simulink model "raibert_controller_1_1"  (R2018b)
settings: Solver=ode15s  StartTime=0.0  StopTime=inf  FixedStep=sample_time  MaxStep=1e-2  RelTol=1e-3
InitFcn:
  | addpath('../common/')
  | colors
  | addpath('functions/')
  | simulation_params
  | mechanical_params
StartFcn:
  | clc
  | tic
StopFcn:
  | stopscript
values from neighbouring files (symbols this model uses):
  sample_time = 1/sample_freq    (= 0.001)    [simulation_params.m]
undefined symbols (not defined in the file or in its folder): ctrl, sm
libraries: powerlib_meascontrol x1
settings Model: Creator=William  LastModifiedBy=akhadke
settings DataIOCC: SaveOutput=off  SaveTime=off
settings OptimizationCC: BlockReduction=off  DefaultParameterBehavior=Inlined  UseFloatMulNetSlope=on  InlineInvariantSignals=on  OptimizeBlockIOStorage=off  BufferReuse=off  GlobalBufferReuse=off  ExpressionFolding=off  LocalBlockOutputs=off  LifeSpan=0.5  SimCompilerOptimization=on  OptimizeDataStoreBuffers=off  BusAssignmentInplaceUpdate=off
settings DebuggingCC: UnderspecifiedInitializationDetection=Classic  MergeDetectMultiDrivingBlocksExec=none  LibraryContextMissingDiagnostic=none
settings HardwareCC: ProdBitPerPointer=32  ProdBitPerSizeT=32  ProdBitPerPtrDiffT=32  ProdLargestAtomicFloat=None  ProdWordSize=32  ProdLongLongMode=on  ProdHWDeviceType=Generic->32-bit x86 compatible
settings ModelReferenceCC: PropagateSignalLabelsOutOfModel=off
settings SFSimCC: SimUseLocalCustomCode=off
settings RTWCC: SystemTargetFile=slrt.tlc  TLCOptions=-axPCModelStackSizeKB=1024  TemplateMakefile=slrt_default_tmf  Description=Simulink Real-Time  RTWUseLocalCustomCode=off  CodeExecutionProfiling=on  RTWCompilerOptimization=on
settings CodeAppCC: MaxIdLength=127  StateflowObjectComments=on
settings TargetCC: CodeReplacementLibrary=XPC_BLAS  ParMdlRefBuildCompliant=on  ConcurrentExecutionCompliant=on  GeneratePreprocessorConditionals=Use local settings  MatFileLogging=on  PreserveStateflowLocalDataDimensions=off  MATLABClassNameForMDSCustomization=xpcAperiodicCustomization
settings SimscapeCC: SimscapeNormalizeSystem=off

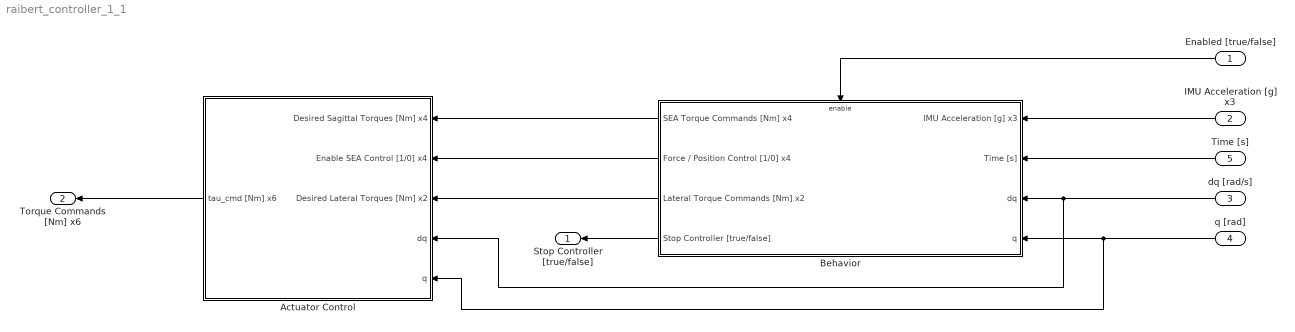
== system raibert_controller_1_1 ==
  Enabled [true/false] : Inport  OutDataTypeStr=boolean  PortDimensions=1  SampleTime=sample_time  Interpolate=off
  IMU Acceleration [g] x3 : Inport  Port=2  OutDataTypeStr=double  PortDimensions=3  SampleTime=[0.001,0]  Interpolate=off
  dq [rad/s] : Inport  Port=3  OutDataTypeStr=double  PortDimensions=13  SampleTime=[0.001,0]  Interpolate=off
  q [rad] : Inport  Port=4  OutDataTypeStr=double  PortDimensions=13  SampleTime=[0.001,0]  Interpolate=off
  Time [s] : Inport  Port=5  OutDataTypeStr=double  PortDimensions=1  SampleTime=sample_time  Interpolate=off
  Actuator Control : Subsystem
  Behavior : Subsystem
  Stop Controller [true/false] : Outport  OutDataTypeStr=boolean  PortDimensions=1  SampleTime=[0.001,0]  OutputWhenDisabled=reset  InitialOutput=[0 0 0 0 0 0]
  Torque Commands [Nm] x6 : Outport  Port=2  OutDataTypeStr=double  PortDimensions=6  SampleTime=[0.001,0]  OutputWhenDisabled=reset  InitialOutput=[0 0 0 0 0 0]
  wires:
  Behavior/2(Force / Position Control [1/0] x4) -> Actuator Control/2(Enable SEA Control [1/0] x4)
  IMU Acceleration [g] x3/1 -> Behavior/1(IMU Acceleration [g] x3)
  Time [s]/1 -> Behavior/2(Time [s])
  Behavior/3(Lateral Torque Commands [Nm] x2) -> Actuator Control/3(Desired Lateral Torques [Nm] x2)
  Behavior/1(SEA Torque Commands [Nm] x4) -> Actuator Control/1(Desired Sagittal Torques [Nm] x4)
  Actuator Control/1(tau_cmd [Nm] x6) -> Torque Commands [Nm] x6/1
  q [rad]/1 -> Actuator Control/5(q), Behavior/4(q)
  dq [rad/s]/1 -> Actuator Control/4(dq), Behavior/3(dq)
  Enabled [true/false]/1 -> Behavior/Enable
  Behavior/4(Stop Controller [true/false]) -> Stop Controller [true/false]/1

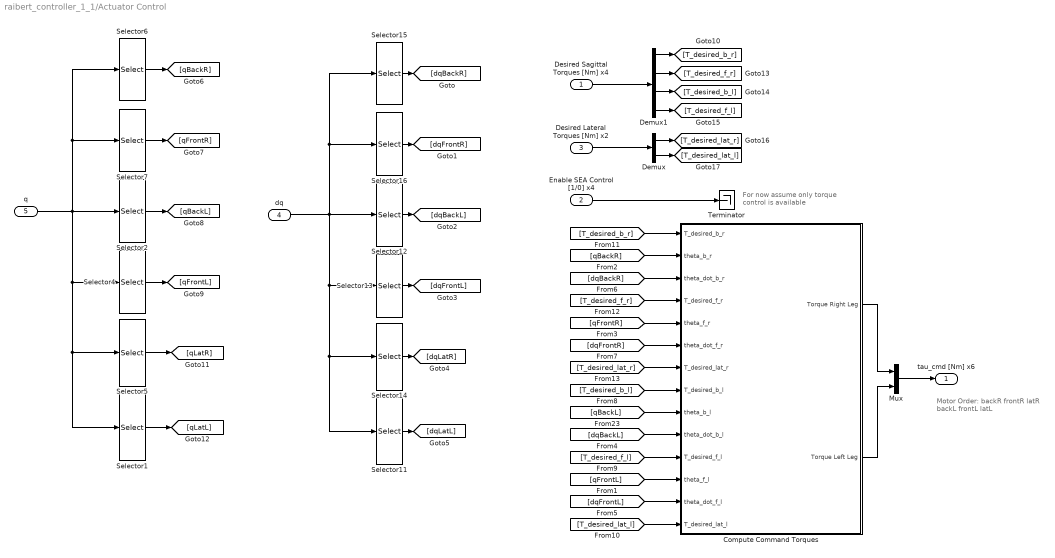
== system raibert_controller_1_1/Actuator Control ==
  note: Motor Order:
      |
      | backR
      | frontR
      | latR
      | backL
      | frontL
      | latL
  note: For now assume only
      | torque control is available
  Desired Sagittal Torques [Nm] x4 : Inport  OutDataTypeStr=double  PortDimensions=4  SampleTime=sample_time
  Enable SEA Control [1/0] x4 : Inport  Port=2  OutDataTypeStr=boolean  PortDimensions=4  SampleTime=sample_time
  Desired Lateral Torques [Nm] x2 : Inport  Port=3  OutDataTypeStr=double  PortDimensions=2  SampleTime=sample_time
  dq : Inport  Port=4  OutDataTypeStr=double  PortDimensions=13  SampleTime=sample_time
  q : Inport  Port=5  OutDataTypeStr=double  PortDimensions=13  SampleTime=sample_time
  Compute Command Torques : Subsystem
  Demux : Demux  Outputs=2
  Demux1 : Demux
  Mux : Mux  Inputs=2
  Selector1 : Selector  InputPortWidth=13  IndexOptions=Index vector (dialog)  Indices=[10]  OutputSizes=1
  Selector11 : Selector  InputPortWidth=13  IndexOptions=Index vector (dialog)  Indices=[10]  OutputSizes=1
  Selector12 : Selector  InputPortWidth=13  IndexOptions=Index vector (dialog)  Indices=[5 6]  OutputSizes=1
  Selector13 : Selector  InputPortWidth=13  IndexOptions=Index vector (dialog)  Indices=[7 8]  OutputSizes=1
  Selector14 : Selector  InputPortWidth=13  IndexOptions=Index vector (dialog)  Indices=[9]  OutputSizes=1
  Selector15 : Selector  InputPortWidth=13  IndexOptions=Index vector (dialog)  Indices=[1 2]  OutputSizes=1
  Selector16 : Selector  InputPortWidth=13  IndexOptions=Index vector (dialog)  Indices=[3 4]  OutputSizes=1
  Selector2 : Selector  InputPortWidth=13  IndexOptions=Index vector (dialog)  Indices=[5 6]  OutputSizes=1
  Selector4 : Selector  InputPortWidth=13  IndexOptions=Index vector (dialog)  Indices=[7 8]  OutputSizes=1
  Selector5 : Selector  InputPortWidth=13  IndexOptions=Index vector (dialog)  Indices=[9]  OutputSizes=1
  Selector6 : Selector  InputPortWidth=13  IndexOptions=Index vector (dialog)  Indices=[1 2]  OutputSizes=1
  Selector7 : Selector  InputPortWidth=13  IndexOptions=Index vector (dialog)  Indices=[3 4]  OutputSizes=1
  Terminator : Terminator
  tau_cmd [Nm] x6 : Outport  OutDataTypeStr=double  PortDimensions=6  InitialOutput=[0 0 0 0 0 0]
  wires:
  Compute Command Torques/2(Torque Left Leg) -> Mux/2
  Compute Command Torques/1(Torque Right Leg) -> Mux/1
  Mux/1 -> tau_cmd [Nm] x6/1
  [T_desired_lat_r] -> Compute Command Torques/7(T_desired_lat_r)
  [T_desired_f_r] -> Compute Command Torques/4(T_desired_f_r)
  [T_desired_b_r] -> Compute Command Torques/1(T_desired_b_r)
  Demux/2 -> [T_desired_lat_l]
  Demux/1 -> [T_desired_lat_r]
  [T_desired_lat_l] -> Compute Command Torques/14(T_desired_lat_l)
  [T_desired_f_l] -> Compute Command Torques/11(T_desired_f_l)
  [T_desired_b_l] -> Compute Command Torques/8(T_desired_b_l)
  Demux1/4 -> [T_desired_f_l]
  Demux1/3 -> [T_desired_b_l]
  Demux1/2 -> [T_desired_f_r]
  Demux1/1 -> [T_desired_b_r]
  Enable SEA Control [1/0] x4/1 -> Terminator/1
  Desired Sagittal Torques [Nm] x4/1 -> Demux1/1
  Desired Lateral Torques [Nm] x2/1 -> Demux/1
  [qBackR] -> Compute Command Torques/2(theta_b_r)
  [dqBackR] -> Compute Command Torques/3(theta_dot_b_r)
  [qFrontR] -> Compute Command Torques/5(theta_f_r)
  [dqFrontR] -> Compute Command Torques/6(theta_dot_f_r)
  [dqFrontL] -> Compute Command Torques/13(theta_dot_f_l)
  [qFrontL] -> Compute Command Torques/12(theta_f_l)
  [qBackL] -> Compute Command Torques/9(theta_b_l)
  [dqBackL] -> Compute Command Torques/10(theta_dot_b_l)
  Selector14/1 -> [dqLatR]
  Selector16/1 -> [dqFrontR]
  Selector7/1 -> [qFrontR]
  q/1 -> Selector2/1, Selector7/1, Selector6/1, Selector4/1, Selector5/1, Selector1/1
  Selector11/1 -> [dqLatL]
  dq/1 -> Selector11/1, Selector14/1, Selector13/1, Selector15/1, Selector16/1, Selector12/1
  Selector6/1 -> [qBackR]
  Selector5/1 -> [qLatR]
  Selector4/1 -> [qFrontL]
  Selector2/1 -> [qBackL]
  Selector12/1 -> [dqBackL]
  Selector1/1 -> [qLatL]
  Selector13/1 -> [dqFrontL]
  Selector15/1 -> [dqBackR]

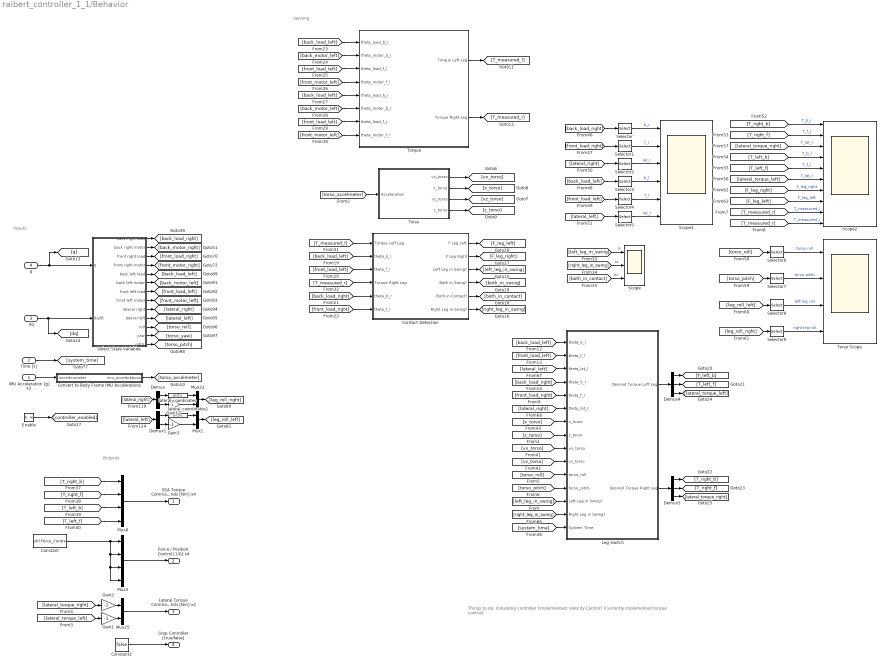
== system raibert_controller_1_1/Behavior ==
  note: Inputs
  note: Sensing
  note: Outputs
  note: Things to do:
      | Initializing controller (implemented)
      | Velocity Control? (Currently implemented torque control)
  IMU Acceleration [g] x3 : Inport  OutDataTypeStr=double  PortDimensions=3  SampleTime=[0.001,0]
  Time [s] : Inport  Port=2  OutDataTypeStr=double  PortDimensions=1  SampleTime=[0.001,0]
  dq : Inport  Port=3  OutDataTypeStr=double  PortDimensions=13  SampleTime=[0.001,0]
  q : Inport  Port=4  OutDataTypeStr=double  PortDimensions=13  SampleTime=[0.001,0]
  Enable : EnablePort  PropagateVarSize=During execution  ShowOutputPort=on
  Constant : Constant  Value=ctrl.Force_Control
  Constant2 : Constant  Value=false
  Contact Detection : Subsystem
  Convert to Body Frame IMU Accelerations : MATLAB Function  TreatAsAtomicUnit=on
  Demux : Demux  Outputs=2
  Demux1 : Demux  Outputs=2
  Demux3 : Demux  Outputs=3
  Demux4 : Demux  Outputs=3
  Gain{1..3,12} (4 alike) : Gain  Gain=-1
  Leg Switch : Subsystem
  Mux1 : Mux  Inputs=2
  Mux22 : Mux  Inputs=2
  Mux25 : Mux  Inputs=2
  Mux3 : Mux
  Mux8 : Mux
  Scope : Scope  NumInputPorts=3
  Scope1 : Scope  NumInputPorts=6
  Scope2 : Scope  NumInputPorts=10
  Select State Variables : Subsystem
  Selector{,1..9} (10 alike) : Selector  InputPortWidth=2  IndexOptions=Index vector (dialog)  Indices=[1]  OutputSizes=1
  Torque : Subsystem
  Torso : Subsystem
  Torso Scope : Scope  NumInputPorts=4
  lateral_coordinates : Fcn  Expr=pi/2-u
  lateral_coordinates1 : Fcn  Expr=pi/2-u
  SEA Torque Commands [Nm] x4 : Outport  OutDataTypeStr=double  PortDimensions=4  SampleTime=[0.001,0]  OutputWhenDisabled=reset  InitialOutput=[0 0 0 0]
  Force / Position Control [1/0] x4 : Outport  Port=2  OutDataTypeStr=boolean  PortDimensions=4  SampleTime=[0.001,0]  OutputWhenDisabled=reset  InitialOutput=[0 0 0 0]
  Lateral Torque Commands [Nm] x2 : Outport  Port=3  OutDataTypeStr=double  PortDimensions=2  SampleTime=[0.001,0]  OutputWhenDisabled=reset  InitialOutput=[0 0]
  Stop Controller [true/false] : Outport  Port=4  OutDataTypeStr=boolean  PortDimensions=1  SampleTime=[0.001,0]  OutputWhenDisabled=reset  InitialOutput=0
  wires:
  [T_measured_r] -> Scope2/10  "T_measured_r"
  [T_measured_r] -> Scope2/9  "T_measured_l"
  [torso_pitch] -> Leg Switch/12(torso_pitch)
  [torso_roll] -> Leg Switch/11(torso_roll)
  [z_torso] -> Leg Switch/8(z_torso)
  [x_torso] -> Leg Switch/7(x_torso)
  [vz_torso] -> Leg Switch/10(vz_torso)
  [vx_torso] -> Leg Switch/9(vx_torso)
  [lateral_right] -> Leg Switch/6(theta_lat_r)
  [lateral_left] -> Leg Switch/3(theta_lat_l)
  [right_leg_in_swing] -> Leg Switch/14(Right Leg in Swing?)
  [F_leg_left] -> Scope2/8  "F_leg_left"
  [F_leg_right] -> Scope2/7  "F_leg_right"
  Contact Detection/2(F Leg Right) -> [F_leg_right]
  Contact Detection/1(F Leg Left) -> [F_leg_left]
  [leg_roll_right] -> Selector9/1
  Selector9/1 -> Torso Scope/4  "right leg roll"
  [leg_roll_left] -> Selector8/1
  Selector8/1 -> Torso Scope/3  "left leg roll"
  [torso_pitch] -> Selector7/1
  Selector7/1 -> Torso Scope/2  "torso pitch"
  Selector6/1 -> Torso Scope/1  "torso roll"
  [torso_roll] -> Selector6/1
  [lateral_torque_left] -> Scope2/6  "T_lat_l"
  [lateral_torque_right] -> Scope2/3  "T_lat_r"
  [T_left_f] -> Scope2/5  "T_f_l"
  [T_left_b] -> Scope2/4  "T_b_l"
  [T_right_f] -> Scope2/2  "T_f_r"
  [T_right_b] -> Scope2/1  "T_b_r"
  [back_load_right] -> Selector/1
  Selector/1 -> Scope1/1  "b_r"
  Selector2/1 -> Scope1/3  "lat_r"
  [back_load_left] -> Selector3/1
  Selector5/1 -> Scope1/6  "lat_l"
  [lateral_left] -> Selector5/1
  [lateral_right] -> Selector2/1
  Selector4/1 -> Scope1/5  "f_l"
  [front_load_left] -> Selector4/1
  Selector3/1 -> Scope1/4  "b_l"
  [front_load_right] -> Selector1/1
  Selector1/1 -> Scope1/2  "f_r"
  Demux3/3 -> [lateral_torque_right]
  Demux3/2 -> [T_right_f]
  Demux3/1 -> [T_right_b]
  Demux4/3 -> [lateral_torque_left]
  [back_motor_left] -> Torque/6(theta_motor_b_r)
  [back_load_left] -> Torque/5(theta_load_b_r)
  [back_motor_left] -> Torque/2(theta_motor_b_l)
  [front_motor_left] -> Torque/8(theta_motor_f_r)
  [back_load_left] -> Torque/1(theta_load_b_l)
  Torque/2(Torque Right Leg) -> [T_measured_r]
  [front_motor_left] -> Torque/4(theta_motor_f_l)
  [front_load_left] -> Torque/7(theta_load_f_r)
  [front_load_left] -> Torque/3(theta_load_f_l)
  Torque/1(Torque Left Leg) -> [T_measured_l]
  [T_left_f] -> Mux8/4
  [T_left_b] -> Mux8/3
  [T_right_f] -> Mux8/2
  [T_right_b] -> Mux8/1
  Leg Switch/2(Desired Torque Right Leg) -> Demux3/1
  Leg Switch/1(Desired Torque Left Leg) -> Demux4/1
  Demux4/1 -> [T_left_b]
  Demux4/2 -> [T_left_f]
  [system_time] -> Leg Switch/15(System Time)
  Contact Detection/4(Both in Swing?) -> [both_in_swing]
  Contact Detection/5(Both in Contact?) -> [both_in_contact]
  Contact Detection/6(Right Leg in Swing?) -> [right_leg_in_swing]
  Contact Detection/3(Left Leg in Swing?) -> [left_leg_in_swing]
  [both_in_contact] -> Scope/3  "bc"
  [right_leg_in_swing] -> Scope/2  "rs"
  [left_leg_in_swing] -> Scope/1  "ls"
  [T_measured_r] -> Contact Detection/4(Torque Right Leg)
  [T_measured_l] -> Contact Detection/1(Torque Left Leg)
  [front_load_right] -> Contact Detection/6(theta_f_r)
  [back_load_right] -> Contact Detection/5(theta_b_r)
  [front_load_left] -> Contact Detection/3(theta_f_l)
  [back_load_left] -> Contact Detection/2(theta_b_l)
  Torso/4(z_torso) -> [z_torso]
  Torso/2(x_torso) -> [x_torso]
  Torso/3(vz_torso) -> [vz_torso]
  Torso/1(vx_torso) -> [vx_torso]
  [left_leg_in_swing] -> Leg Switch/13("Left Leg in Swing? ")
  Constant/1 -> Mux3/1, Mux3/2, Mux3/3, Mux3/4
  [front_load_left] -> Leg Switch/2(theta_f_l)
  [back_load_left] -> Leg Switch/1(theta_b_l)
  [front_load_right] -> Leg Switch/5(theta_f_r)
  [back_load_right] -> Leg Switch/4(theta_b_r)
  [torso_accelmeter] -> Torso/1(Acceleration)
  IMU Acceleration [g] x3/1 -> Convert to Body Frame IMU Accelerations/1(accelerometer)
  Convert to Body Frame IMU Accelerations/1(imu_accelerations) -> [torso_accelmeter]
  Enable/1 -> [controller_enabled]
  Demux1/2 -> Gain3/1
  lateral_coordinates1/1 -> Mux1/1
  Gain3/1 -> Mux1/2
  Mux1/1 -> [leg_roll_left]
  Demux1/1 -> lateral_coordinates1/1
  [lateral_left] -> Demux1/1
  [lateral_right] -> Demux/1
  Select State Variables/9(lateral right) -> [lateral_right]
  Select State Variables/10(lateral left) -> [lateral_left]
  Select State Variables/11(roll) -> [torso_roll]
  Select State Variables/12(yaw) -> [torso_yaw]
  Select State Variables/13(pitch) -> [torso_pitch]
  Select State Variables/8(front left motor) -> [front_motor_left]
  Select State Variables/7(front left load) -> [front_load_left]
  Select State Variables/6(back left motor) -> [back_motor_left]
  Select State Variables/5(back left load) -> [back_load_left]
  Select State Variables/4(front right motor) -> [front_motor_right]
  Select State Variables/3(front right load) -> [front_load_right]
  Select State Variables/2(back right motor) -> [back_motor_right]
  Select State Variables/1(back right load) -> [back_load_right]
  dq/1 -> Select State Variables/2(dq/dt), [dq]
  Constant2/1 -> Stop Controller [true/false]/1
  Gain1/1 -> Mux25/2
  Mux25/1 -> Lateral Torque Commands [Nm] x2/1
  Gain2/1 -> Mux25/1
  Mux3/1 -> Force / Position Control [1/0] x4/1
  Mux8/1 -> SEA Torque Commands [Nm] x4/1
  [lateral_torque_left] -> Gain1/1
  q/1 -> Select State Variables/1(q), [q]
  [lateral_torque_right] -> Gain2/1
  Demux/1 -> lateral_coordinates/1
  Mux22/1 -> [leg_roll_right]
  Gain12/1 -> Mux22/2
  lateral_coordinates/1 -> Mux22/1
  Demux/2 -> Gain12/1
  Time [s]/1 -> [system_time]

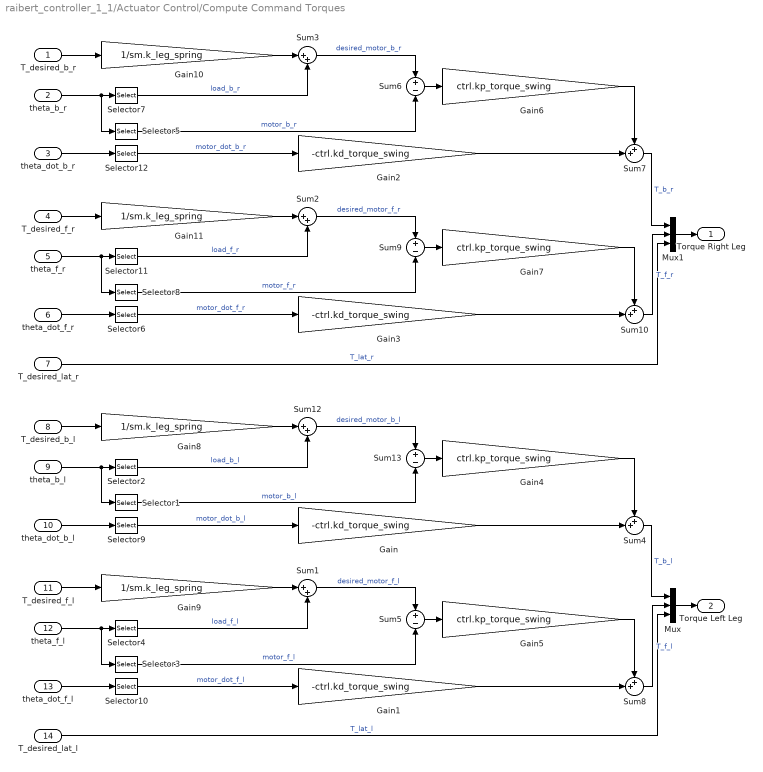
== system raibert_controller_1_1/Actuator Control/Compute Command Torques ==
  T_desired_b_r : Inport
  theta_b_r : Inport  Port=2
  theta_dot_b_r : Inport  Port=3
  T_desired_f_r : Inport  Port=4
  theta_f_r : Inport  Port=5
  theta_dot_f_r : Inport  Port=6
  T_desired_lat_r : Inport  Port=7
  T_desired_b_l : Inport  Port=8
  theta_b_l : Inport  Port=9
  theta_dot_b_l : Inport  Port=10
  T_desired_f_l : Inport  Port=11
  theta_f_l : Inport  Port=12
  theta_dot_f_l : Inport  Port=13
  T_desired_lat_l : Inport  Port=14
  Gain{,1..3} (4 alike) : Gain  Gain=-ctrl.kd_torque_swing
  Gain{8..11} (4 alike) : Gain  Gain=1/sm.k_leg_spring
  Gain{4..7} (4 alike) : Gain  Gain=ctrl.kp_torque_swing
  Mux : Mux  Inputs=3
  Mux1 : Mux  Inputs=3
  Selector{1,3,5..6,8..10,12} (8 alike) : Selector  InputPortWidth=2  IndexOptions=Index vector (dialog)  Indices=[2]  OutputSizes=1
  Selector{2,4,7,11} (4 alike) : Selector  InputPortWidth=2  IndexOptions=Index vector (dialog)  Indices=[1]  OutputSizes=1
  Sum{1..3,12} (4 alike) : Sum  Inputs=|++
  Sum{4,7..8,10} (4 alike) : Sum  Inputs=++|
  Sum{5..6,9,13} (4 alike) : Sum  Inputs=+-
  Torque Right Leg : Outport
  Torque Left Leg : Outport  Port=2
  wires:
  Sum9/1 -> Gain7/1
  theta_f_r/1 -> Selector11/1, Selector8/1
  Selector8/1 -> Sum9/2  "motor_f_r"
  T_desired_f_r/1 -> Gain11/1
  Gain11/1 -> Sum2/1
  Selector5/1 -> Sum6/2  "motor_b_r"
  theta_dot_b_r/1 -> Selector12/1
  Gain3/1 -> Sum10/2
  Selector12/1 -> Gain2/1  "motor_dot_b_r"
  Gain6/1 -> Sum7/1
  Gain2/1 -> Sum7/2
  Mux1/1 -> Torque Right Leg/1
  Selector6/1 -> Gain3/1  "motor_dot_f_r"
  Sum3/1 -> Sum6/1  "desired_motor_b_r"
  T_desired_lat_r/1 -> Mux1/3  "T_lat_r"
  T_desired_b_r/1 -> Gain10/1
  theta_b_r/1 -> Selector7/1, Selector5/1
  theta_dot_f_r/1 -> Selector6/1
  Sum2/1 -> Sum9/1  "desired_motor_f_r"
  Gain10/1 -> Sum3/1
  Gain7/1 -> Sum10/1
  Selector7/1 -> Sum3/2  "load_b_r"
  Sum7/1 -> Mux1/1  "T_b_r"
  Sum6/1 -> Gain6/1
  Selector11/1 -> Sum2/2  "load_f_r"
  Sum10/1 -> Mux1/2  "T_f_r"
  T_desired_lat_l/1 -> Mux/3  "T_lat_l"
  Sum8/1 -> Mux/2  "T_f_l"
  T_desired_f_l/1 -> Gain9/1
  theta_f_l/1 -> Selector4/1, Selector3/1
  Sum1/1 -> Sum5/1  "desired_motor_f_l"
  Selector3/1 -> Sum5/2  "motor_f_l"
  Gain9/1 -> Sum1/1
  Gain1/1 -> Sum8/2
  theta_dot_f_l/1 -> Selector10/1
  Selector10/1 -> Gain1/1  "motor_dot_f_l"
  Gain5/1 -> Sum8/1
  Selector4/1 -> Sum1/2  "load_f_l"
  Sum5/1 -> Gain5/1
  Gain4/1 -> Sum4/1
  Gain/1 -> Sum4/2
  Sum13/1 -> Gain4/1
  Sum12/1 -> Sum13/1  "desired_motor_b_l"
  Gain8/1 -> Sum12/1
  T_desired_b_l/1 -> Gain8/1
  theta_dot_b_l/1 -> Selector9/1
  Selector9/1 -> Gain/1  "motor_dot_b_l"
  theta_b_l/1 -> Selector2/1, Selector1/1
  Selector2/1 -> Sum12/2  "load_b_l"
  Selector1/1 -> Sum13/2  "motor_b_l"
  Sum4/1 -> Mux/1  "T_b_l"
  Mux/1 -> Torque Left Leg/1

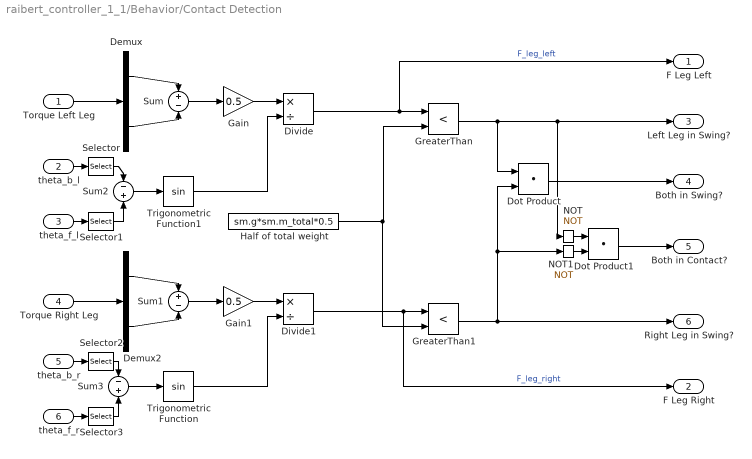
== system raibert_controller_1_1/Behavior/Contact Detection ==
  Torque Left Leg : Inport
  theta_b_l : Inport  Port=2
  theta_f_l : Inport  Port=3
  Torque Right Leg : Inport  Port=4
  theta_b_r : Inport  Port=5
  theta_f_r : Inport  Port=6
  Demux : Demux  Outputs=2
  Demux2 : Demux  Outputs=2
  Divide : Product  Inputs=*/
  Divide1 : Product  Inputs=*/
  Dot Product : DotProduct  InputSameDT=on  OutDataTypeStr=Inherit: Inherit via internal rule
  Dot Product1 : DotProduct  InputSameDT=on  OutDataTypeStr=Inherit: Inherit via internal rule
  Gain : Gain  Gain=0.5
  Gain1 : Gain  Gain=0.5
  GreaterThan : RelationalOperator  Operator=<  OutDataTypeStr=boolean  RndMeth=Simplest
  GreaterThan1 : RelationalOperator  Operator=<  OutDataTypeStr=boolean  RndMeth=Simplest
  Half of total weight : Constant  Value=sm.g*sm.m_total*0.5
  NOT : Logic  Operator=NOT  IconShape=distinctive  AllPortsSameDT=off  OutDataTypeStr=boolean
  NOT1 : Logic  Operator=NOT  IconShape=distinctive  AllPortsSameDT=off  OutDataTypeStr=boolean
  Selector{,1..3} (4 alike) : Selector  InputPortWidth=2  IndexOptions=Index vector (dialog)  Indices=[1]  OutputSizes=1
  Sum : Sum  Inputs=+-
  Sum1 : Sum  Inputs=+-
  Sum2 : Sum  Inputs=-+
  Sum3 : Sum  Inputs=-+
  Trigonometric Function : Trigonometry
  Trigonometric Function1 : Trigonometry
  F Leg Left : Outport
  F Leg Right : Outport  Port=2
  Left Leg in Swing? : Outport  Port=3
  Both in Swing? : Outport  Port=4
  Both in Contact? : Outport  Port=5
  Right Leg in Swing? : Outport  Port=6
  wires:
  Selector3/1 -> Sum3/2
  Selector2/1 -> Sum3/1
  Selector1/1 -> Sum2/2
  Selector/1 -> Sum2/1
  NOT1/1 -> Dot Product1/2
  NOT/1 -> Dot Product1/1
  Dot Product1/1 -> Both in Contact?/1
  Dot Product/1 -> Both in Swing?/1
  GreaterThan1/1 -> Right Leg in Swing?/1, Dot Product/2, NOT1/1
  GreaterThan/1 -> Left Leg in Swing?/1, NOT/1, Dot Product/1
  Half of total weight/1 -> GreaterThan/2, GreaterThan1/2
  Divide1/1 -> GreaterThan1/1, F Leg Right/1  "F_leg_right"
  Divide/1 -> GreaterThan/1, F Leg Left/1  "F_leg_left"
  Trigonometric Function/1 -> Divide1/2
  Gain1/1 -> Divide1/1
  Trigonometric Function1/1 -> Divide/2
  Gain/1 -> Divide/1
  Sum2/1 -> Trigonometric Function1/1
  Sum3/1 -> Trigonometric Function/1
  theta_b_r/1 -> Selector2/1
  theta_f_r/1 -> Selector3/1
  theta_b_l/1 -> Selector/1
  theta_f_l/1 -> Selector1/1
  Sum1/1 -> Gain1/1
  Sum/1 -> Gain/1
  Demux2/2 -> Sum1/2
  Demux2/1 -> Sum1/1
  Torque Right Leg/1 -> Demux2/1
  Demux/2 -> Sum/2
  Demux/1 -> Sum/1
  Torque Left Leg/1 -> Demux/1

== system raibert_controller_1_1/Behavior/Leg Switch ==
  theta_b_l : Inport
  theta_f_l : Inport  Port=2
  theta_lat_l : Inport  Port=3
  theta_b_r : Inport  Port=4
  theta_f_r : Inport  Port=5
  theta_lat_r : Inport  Port=6
  x_torso : Inport  Port=7
  z_torso : Inport  Port=8
  vx_torso : Inport  Port=9
  vz_torso : Inport  Port=10
  torso_roll : Inport  Port=11
  torso_pitch : Inport  Port=12
  "Left Leg in Swing? " : Inport  Port=13
  Right Leg in Swing? : Inport  Port=14
  System Time : Inport  Port=15
  Initialization Controller : Subsystem
  Logical Operator : Logic  AllPortsSameDT=off  OutDataTypeStr=boolean
  NOT : Logic  Operator=NOT  IconShape=distinctive  AllPortsSameDT=off  OutDataTypeStr=boolean
  Raibert : Subsystem
  Sum : Sum  Inputs=|++
  Sum1 : Sum  Inputs=|++
  Desired Torque Left Leg : Outport  SampleTime=[0.001, 0]
  Desired Torque Right Leg : Outport  Port=2  SampleTime=[0.001 0]
  wires:
  vz_torso/1 -> Raibert/10(vz_torso)
  torso_roll/1 -> Raibert/11(torso_roll)
  torso_pitch/1 -> Raibert/12(torso_pitch)
  vx_torso/1 -> Raibert/9(vx_torso)
  z_torso/1 -> Raibert/8(z_torso)
  x_torso/1 -> Raibert/7(x_torso)
  Initialization Controller/2(Desired Torque Right Leg) -> Sum1/2
  Initialization Controller/1(Desired Torque Left Leg) -> Sum/2
  Sum1/1 -> Desired Torque Right Leg/1
  Sum/1 -> Desired Torque Left Leg/1
  theta_lat_r/1 -> Initialization Controller/6(theta_lat_r)
  theta_lat_l/1 -> Initialization Controller/3(theta_lat_l)
  NOT/1 -> Raibert/Enable
  Logical Operator/1 -> NOT/1, Initialization Controller/Enable
  Right Leg in Swing?/1 -> Logical Operator/1
  Raibert/2(Desired Torque Right Leg) -> Sum1/1
  Raibert/1(Desired Torque Left Leg) -> Sum/1
  theta_f_r/1 -> Raibert/6(theta_f_r), Initialization Controller/5(theta_f_r)
  theta_b_r/1 -> Raibert/5(theta_b_r), Initialization Controller/4(theta_b_r)
  theta_f_l/1 -> Raibert/4(theta_f_l), Initialization Controller/2(theta_f_l)
  theta_b_l/1 -> Raibert/3(theta_b_l), Initialization Controller/1(theta_b_l)
  System Time/1 -> Raibert/2(System Time)
  "Left Leg in Swing? "/1 -> Logical Operator/2, Raibert/1(Left Leg in Swing?)

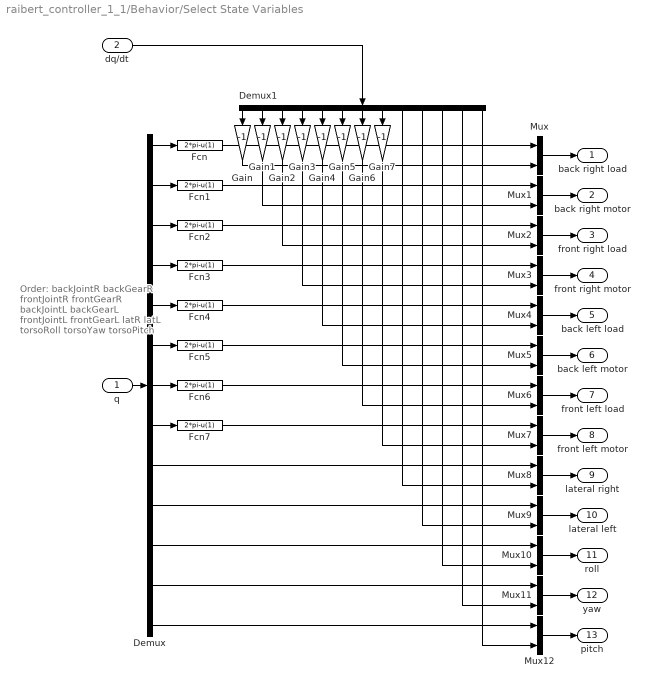
== system raibert_controller_1_1/Behavior/Select State Variables ==
  note: Order:
      |
      | backJointR
      | backGearR
      | frontJointR
      | frontGearR
      |
      | backJointL
      | backGearL
      | frontJointL
      | frontGearL
      |
      | latR
      | latL
      |
      | torsoRoll
      | torsoYaw
      | torsoPitch
  q : Inport
  dq/dt : Inport  Port=2
  Demux : Demux  Outputs=13
  Demux1 : Demux  Outputs=13
  Fcn{,1..7} (8 alike) : Fcn  Expr=2*pi-u(1)
  Gain{,1..7} (8 alike) : Gain  Gain=-1
  Mux{,1..12} (13 alike) : Mux  Inputs=2
  back right load : Outport
  back right motor : Outport  Port=2
  front right load : Outport  Port=3
  front right motor : Outport  Port=4
  back left load : Outport  Port=5
  back left motor : Outport  Port=6
  front left load : Outport  Port=7
  front left motor : Outport  Port=8
  lateral right : Outport  Port=9
  lateral left : Outport  Port=10
  roll : Outport  Port=11
  yaw : Outport  Port=12
  pitch : Outport  Port=13
  wires:
  Gain7/1 -> Mux7/2
  Gain6/1 -> Mux6/2
  Gain5/1 -> Mux5/2
  Gain4/1 -> Mux4/2
  Gain3/1 -> Mux3/2
  Gain2/1 -> Mux2/2
  Gain1/1 -> Mux1/2
  Gain/1 -> Mux/2
  Demux/9 -> Mux8/1
  Fcn7/1 -> Mux7/1
  Fcn6/1 -> Mux6/1
  Fcn5/1 -> Mux5/1
  Fcn4/1 -> Mux4/1
  Fcn3/1 -> Mux3/1
  Fcn2/1 -> Mux2/1
  Fcn1/1 -> Mux1/1
  Fcn/1 -> Mux/1
  dq/dt/1 -> Demux1/1
  Demux1/13 -> Mux12/2
  Demux1/12 -> Mux11/2
  Demux1/11 -> Mux10/2
  Demux1/10 -> Mux9/2
  Demux1/9 -> Mux8/2
  Demux1/8 -> Gain7/1
  Demux1/7 -> Gain6/1
  Demux1/6 -> Gain5/1
  Demux1/5 -> Gain4/1
  Demux1/4 -> Gain3/1
  Demux1/3 -> Gain2/1
  Demux1/2 -> Gain1/1
  Demux/13 -> Mux12/1
  Demux/12 -> Mux11/1
  Demux/11 -> Mux10/1
  Demux/10 -> Mux9/1
  Demux/8 -> Fcn7/1
  Demux/7 -> Fcn6/1
  Demux/6 -> Fcn5/1
  Demux/5 -> Fcn4/1
  Demux/4 -> Fcn3/1
  Demux/3 -> Fcn2/1
  Demux/2 -> Fcn1/1
  Demux1/1 -> Gain/1
  Demux/1 -> Fcn/1
  Mux11/1 -> yaw/1
  Mux10/1 -> roll/1
  Mux7/1 -> front left motor/1
  Mux6/1 -> front left load/1
  Mux3/1 -> front right motor/1
  Mux2/1 -> front right load/1
  Mux12/1 -> pitch/1
  Mux9/1 -> lateral left/1
  Mux8/1 -> lateral right/1
  Mux5/1 -> back left motor/1
  Mux4/1 -> back left load/1
  Mux1/1 -> back right motor/1
  Mux/1 -> back right load/1
  q/1 -> Demux/1

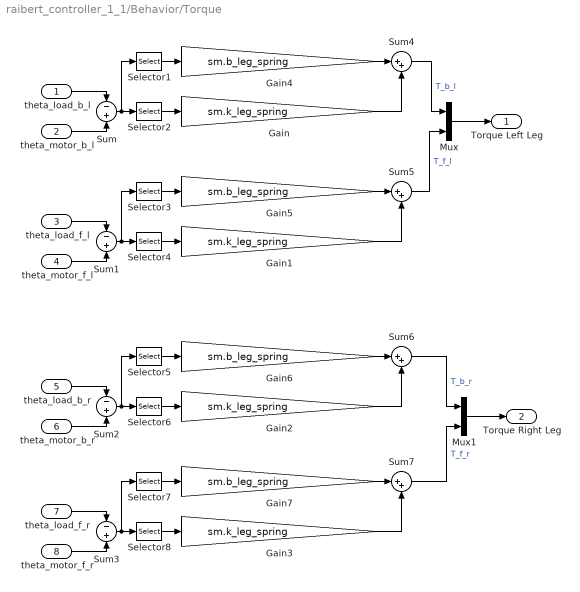
== system raibert_controller_1_1/Behavior/Torque ==
  theta_load_b_l : Inport
  theta_motor_b_l : Inport  Port=2
  theta_load_f_l : Inport  Port=3
  theta_motor_f_l : Inport  Port=4
  theta_load_b_r : Inport  Port=5
  theta_motor_b_r : Inport  Port=6
  theta_load_f_r : Inport  Port=7
  theta_motor_f_r : Inport  Port=8
  Gain{,1..3} (4 alike) : Gain  Gain=sm.k_leg_spring
  Gain{4..7} (4 alike) : Gain  Gain=sm.b_leg_spring
  Mux : Mux  Inputs=2
  Mux1 : Mux  Inputs=2
  Selector{1,3,5,7} (4 alike) : Selector  InputPortWidth=2  IndexOptions=Index vector (dialog)  Indices=[2]  OutputSizes=1
  Selector{2,4,6,8} (4 alike) : Selector  InputPortWidth=2  IndexOptions=Index vector (dialog)  Indices=[1]  OutputSizes=1
  Sum{,1..3} (4 alike) : Sum  Inputs=-+
  Sum{4..7} (4 alike) : Sum  Inputs=|++
  Torque Left Leg : Outport
  Torque Right Leg : Outport  Port=2
  wires:
  Selector8/1 -> Gain3/1
  Selector7/1 -> Gain7/1
  Sum3/1 -> Selector8/1, Selector7/1
  Selector6/1 -> Gain2/1
  Selector5/1 -> Gain6/1
  Sum2/1 -> Selector5/1, Selector6/1
  Selector3/1 -> Gain5/1
  Selector4/1 -> Gain1/1
  Sum1/1 -> Selector3/1, Selector4/1
  Selector1/1 -> Gain4/1
  Selector2/1 -> Gain/1
  Sum/1 -> Selector2/1, Selector1/1
  Sum7/1 -> Mux1/2  "T_f_r"
  Gain7/1 -> Sum7/1
  Gain3/1 -> Sum7/2
  Sum6/1 -> Mux1/1  "T_b_r"
  Gain6/1 -> Sum6/1
  Gain2/1 -> Sum6/2
  Sum5/1 -> Mux/2  "T_f_l"
  Gain5/1 -> Sum5/1
  Sum4/1 -> Mux/1  "T_b_l"
  Gain4/1 -> Sum4/1
  theta_motor_f_r/1 -> Sum3/2
  theta_load_f_r/1 -> Sum3/1
  Mux1/1 -> Torque Right Leg/1
  theta_motor_b_r/1 -> Sum2/2
  theta_load_b_r/1 -> Sum2/1
  Mux/1 -> Torque Left Leg/1
  theta_load_f_l/1 -> Sum1/1
  theta_motor_f_l/1 -> Sum1/2
  Gain1/1 -> Sum5/2
  Gain/1 -> Sum4/2
  theta_load_b_l/1 -> Sum/1
  theta_motor_b_l/1 -> Sum/2

== system raibert_controller_1_1/Behavior/Torso ==
  note: Things to do:
      | Add filtering?
  Acceleration : Inport
  "Integrator, Second-Order" : SecondOrderIntegrator  ICX=0
  "Integrator, Second-Order1" : SecondOrderIntegrator  ICX=sm.initial_com_height
  x : Selector  InputPortWidth=3  IndexOptions=Index vector (dialog)  Indices=[1]  OutputSizes=1
  z : Selector  InputPortWidth=3  IndexOptions=Index vector (dialog)  Indices=[3]  OutputSizes=1
  vx_torso : Outport
  x_torso : Outport  Port=2
  vz_torso : Outport  Port=3
  z_torso : Outport  Port=4
  wires:
  "Integrator, Second-Order1"/1 -> z_torso/1
  "Integrator, Second-Order"/1 -> x_torso/1
  "Integrator, Second-Order"/2 -> vx_torso/1
  "Integrator, Second-Order1"/2 -> vz_torso/1
  z/1 -> "Integrator, Second-Order1"/1
  x/1 -> "Integrator, Second-Order"/1
  Acceleration/1 -> x/1, z/1

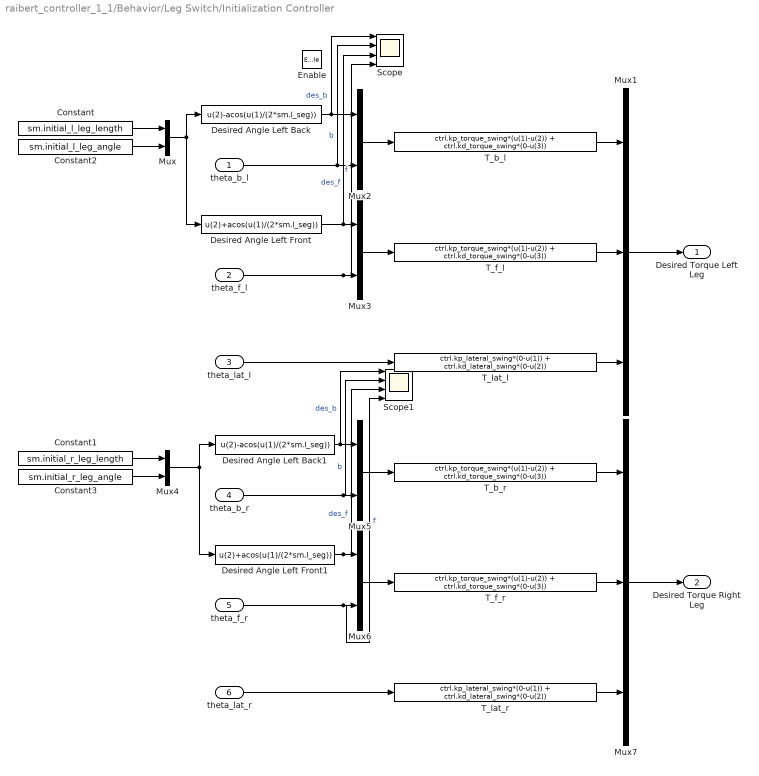
== system raibert_controller_1_1/Behavior/Leg Switch/Initialization Controller ==
  theta_b_l : Inport
  theta_f_l : Inport  Port=2
  theta_lat_l : Inport  Port=3
  theta_b_r : Inport  Port=4
  theta_f_r : Inport  Port=5
  theta_lat_r : Inport  Port=6
  Enable : EnablePort  StatesWhenEnabling=reset  PropagateVarSize=During execution
  Constant : Constant  Value=sm.initial_l_leg_length
  Constant1 : Constant  Value=sm.initial_r_leg_length
  Constant2 : Constant  Value=sm.initial_l_leg_angle
  Constant3 : Constant  Value=sm.initial_r_leg_angle
  Desired Angle Left Back : Fcn  Expr=u(2)-acos(u(1)/(2*sm.l_seg))
  Desired Angle Left Back1 : Fcn  Expr=u(2)-acos(u(1)/(2*sm.l_seg))
  Desired Angle Left Front : Fcn  Expr=u(2)+acos(u(1)/(2*sm.l_seg))
  Desired Angle Left Front1 : Fcn  Expr=u(2)+acos(u(1)/(2*sm.l_seg))
  Mux{,2..6} (6 alike) : Mux  Inputs=2
  Mux1 : Mux  Inputs=3
  Mux7 : Mux  Inputs=3
  Scope : Scope  NumInputPorts=4
  Scope1 : Scope  NumInputPorts=4
  T_b_l : Fcn  Expr=ctrl.kp_torque_swing*(u(1)-u(2)) + ctrl.kd_torque_swing*(0-u(3))
  T_b_r : Fcn  Expr=ctrl.kp_torque_swing*(u(1)-u(2)) + ctrl.kd_torque_swing*(0-u(3))
  T_f_l : Fcn  Expr=ctrl.kp_torque_swing*(u(1)-u(2)) + ctrl.kd_torque_swing*(0-u(3))
  T_f_r : Fcn  Expr=ctrl.kp_torque_swing*(u(1)-u(2)) + ctrl.kd_torque_swing*(0-u(3))
  T_lat_l : Fcn  Expr=ctrl.kp_lateral_swing*(0-u(1)) + ctrl.kd_lateral_swing*(0-u(2))
  T_lat_r : Fcn  Expr=ctrl.kp_lateral_swing*(0-u(1)) + ctrl.kd_lateral_swing*(0-u(2))
  Desired Torque Left Leg : Outport  InitialOutput=[0 0 0]
  Desired Torque Right Leg : Outport  Port=2  InitialOutput=[0 0 0]
  wires:
  theta_b_r/1 -> Mux5/2, Scope1/2  "b"
  theta_f_r/1 -> Mux6/2, Scope1/4  "f"
  Desired Angle Left Front1/1 -> Mux6/1, Scope1/3  "des_f"
  Desired Angle Left Back1/1 -> Mux5/1, Scope1/1  "des_b"
  Mux1/1 -> Desired Torque Left Leg/1
  Mux7/1 -> Desired Torque Right Leg/1
  T_lat_r/1 -> Mux7/3
  T_f_r/1 -> Mux7/2
  T_b_r/1 -> Mux7/1
  T_lat_l/1 -> Mux1/3
  T_f_l/1 -> Mux1/2
  T_b_l/1 -> Mux1/1
  Constant3/1 -> Mux4/2
  Constant1/1 -> Mux4/1
  Mux6/1 -> T_f_r/1
  Mux5/1 -> T_b_r/1
  theta_lat_r/1 -> T_lat_r/1
  Mux4/1 -> Desired Angle Left Back1/1, Desired Angle Left Front1/1
  Desired Angle Left Front/1 -> Mux3/1, Scope/3  "des_f"
  Mux3/1 -> T_f_l/1
  theta_f_l/1 -> Mux3/2, Scope/4  "f"
  Mux2/1 -> T_b_l/1
  theta_b_l/1 -> Mux2/2, Scope/2  "b"
  Desired Angle Left Back/1 -> Mux2/1, Scope/1  "des_b"
  Constant2/1 -> Mux/2
  Constant/1 -> Mux/1
  Mux/1 -> Desired Angle Left Back/1, Desired Angle Left Front/1
  theta_lat_l/1 -> T_lat_l/1

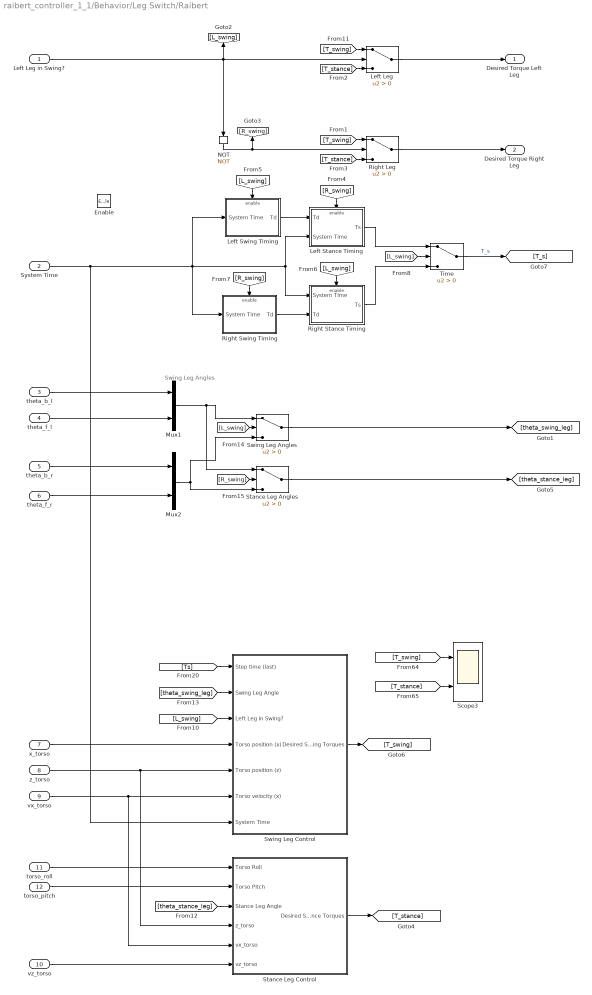
== system raibert_controller_1_1/Behavior/Leg Switch/Raibert ==
  note: Swing Leg Angles
  Left Leg in Swing? : Inport
  System Time : Inport  Port=2
  theta_b_l : Inport  Port=3
  theta_f_l : Inport  Port=4
  theta_b_r : Inport  Port=5
  theta_f_r : Inport  Port=6
  x_torso : Inport  Port=7
  z_torso : Inport  Port=8
  vx_torso : Inport  Port=9
  vz_torso : Inport  Port=10
  torso_roll : Inport  Port=11
  torso_pitch : Inport  Port=12
  Enable : EnablePort  StatesWhenEnabling=reset  PropagateVarSize=During execution
  Left Leg : Switch  Criteria=u2 > Threshold
  Left Stance Timing : Subsystem
  Left Swing Timing : Subsystem
  Mux1 : Mux  Inputs=2
  Mux2 : Mux  Inputs=2
  NOT : Logic  Operator=NOT  IconShape=distinctive  AllPortsSameDT=off  OutDataTypeStr=boolean
  Right Leg : Switch  Criteria=u2 > Threshold
  Right Stance Timing : Subsystem
  Right Swing Timing : Subsystem
  Scope3 : Scope  NumInputPorts=2
  Stance Leg Angles : Switch  Criteria=u2 > Threshold
  Stance Leg Control : Subsystem  TreatAsAtomicUnit=on
  Swing Leg Angles : Switch  Criteria=u2 > Threshold
  Swing Leg Control : Subsystem  TreatAsAtomicUnit=on
  Time : Switch  Criteria=u2 > Threshold
  Desired Torque Left Leg : Outport  InitialOutput=[0 0 0]
  Desired Torque Right Leg : Outport  Port=2  InitialOutput=[0 0 0]
  wires:
  Swing Leg Control/1(Desired Swing Torques) -> [T_swing]
  torso_pitch/1 -> Stance Leg Control/2(Torso Pitch)
  [T_stance] -> Scope3/2
  System Time/1 -> Right Swing Timing/1(System Time), Right Stance Timing/1(System Time), Left Stance Timing/2(System Time), Left Swing Timing/1(System Time), Swing Leg Control/7(System Time)
  [theta_swing_leg] -> Swing Leg Control/2(Swing Leg Angle)
  [theta_stance_leg] -> Stance Leg Control/3(Stance Leg Angle)
  [T_swing] -> Scope3/1
  z_torso/1 -> Swing Leg Control/5(Torso position (z)), Stance Leg Control/4(z_torso)
  x_torso/1 -> Swing Leg Control/4(Torso position (x))
  [Ts] -> Swing Leg Control/1(Step time (last))
  Stance Leg Control/1(Desired Stance Torques) -> [T_stance]
  vz_torso/1 -> Stance Leg Control/6(vz_torso)
  [L_swing] -> Swing Leg Control/3(Left Leg in Swing?)
  torso_roll/1 -> Stance Leg Control/1(Torso Roll)
  vx_torso/1 -> Swing Leg Control/6(Torso velocity (x)), Stance Leg Control/5(vx_torso)
  Right Swing Timing/1(Td) -> Right Stance Timing/2(Td)
  theta_b_l/1 -> Mux1/1
  Mux1/1 -> Swing Leg Angles/1, Stance Leg Angles/1
  Left Stance Timing/1(Ts) -> Time/1
  [R_swing] -> Stance Leg Angles/2
  [T_swing] -> Left Leg/1
  Stance Leg Angles/1 -> [theta_stance_leg]
  Mux2/1 -> Swing Leg Angles/3, Stance Leg Angles/3
  Left Swing Timing/1(Td) -> Left Stance Timing/1(Td)
  [T_swing] -> Right Leg/1
  theta_f_r/1 -> Mux2/2
  [R_swing] -> Left Stance Timing/Enable
  Time/1 -> [T_s]  "T_s"
  [T_stance] -> Left Leg/3
  [L_swing] -> Swing Leg Angles/2
  theta_f_l/1 -> Mux1/2
  [L_swing] -> Left Swing Timing/Enable
  Right Stance Timing/1(Ts) -> Time/3
  Left Leg in Swing?/1 -> [L_swing], Left Leg/2, NOT/1
  NOT/1 -> Right Leg/2, [R_swing]
  [R_swing] -> Right Swing Timing/Enable
  theta_b_r/1 -> Mux2/1
  Right Leg/1 -> Desired Torque Right Leg/1
  [L_swing] -> Time/2
  Left Leg/1 -> Desired Torque Left Leg/1
  Swing Leg Angles/1 -> [theta_swing_leg]
  [L_swing] -> Right Stance Timing/Enable
  [T_stance] -> Right Leg/3

== system raibert_controller_1_1/Behavior/Leg Switch/Raibert/Left Stance Timing ==
  Td : Inport
  System Time : Inport  Port=2
  Enable : EnablePort
  Memory : Memory
  Sum : Sum  Inputs=|+-
  Ts : Outport
  wires:
  Sum/1 -> Memory/1
  Memory/1 -> Ts/1
  Td/1 -> Sum/2
  System Time/1 -> Sum/1

== system raibert_controller_1_1/Behavior/Leg Switch/Raibert/Left Swing Timing ==
  System Time : Inport
  Enable : EnablePort
  Td : Outport
  wires:
  System Time/1 -> Td/1

== system raibert_controller_1_1/Behavior/Leg Switch/Raibert/Right Stance Timing ==
  System Time : Inport
  Td : Inport  Port=2
  Enable : EnablePort
  Memory : Memory
  Sum : Sum  Inputs=|+-
  Ts : Outport
  wires:
  Sum/1 -> Memory/1
  Memory/1 -> Ts/1
  Td/1 -> Sum/2
  System Time/1 -> Sum/1

== system raibert_controller_1_1/Behavior/Leg Switch/Raibert/Right Swing Timing ==
  System Time : Inport
  Enable : EnablePort
  Td : Outport
  wires:
  System Time/1 -> Td/1

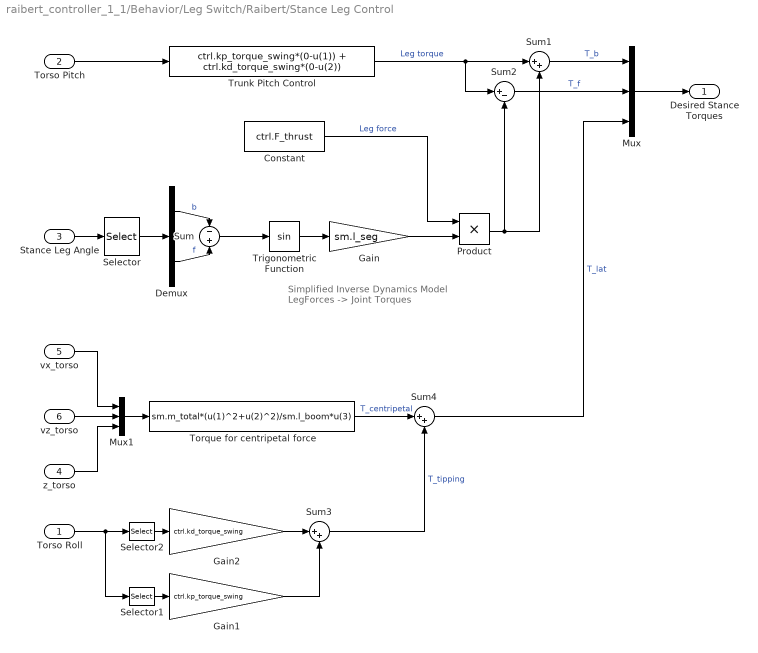
== system raibert_controller_1_1/Behavior/Leg Switch/Raibert/Stance Leg Control ==
  note: Simplified Inverse Dynamics Model
      | LegForces -> Joint Torques
  Torso Roll : Inport
  Torso Pitch : Inport  Port=2
  Stance Leg Angle : Inport  Port=3
  z_torso : Inport  Port=4
  vx_torso : Inport  Port=5
  vz_torso : Inport  Port=6
  Constant : Constant  Value=ctrl.F_thrust
  Demux : Demux  Outputs=2
  Gain : Gain  Gain=sm.l_seg
  Gain1 : Gain  Gain=ctrl.kp_torque_swing
  Gain2 : Gain  Gain=ctrl.kd_torque_swing
  Mux : Mux  Inputs=3
  Mux1 : Mux  Inputs=3
  Product : Product
  Selector : Selector  InputPortWidth=4  IndexOptions=Index vector (dialog)  Indices=[1 3]  OutputSizes=1
  Selector1 : Selector  InputPortWidth=2  IndexOptions=Index vector (dialog)  Indices=[1]  OutputSizes=1
  Selector2 : Selector  InputPortWidth=2  IndexOptions=Index vector (dialog)  Indices=[2]  OutputSizes=1
  Sum : Sum  Inputs=-+
  Sum1 : Sum  Inputs=|++
  Sum2 : Sum  Inputs=|+-
  Sum3 : Sum  Inputs=|++
  Sum4 : Sum  Inputs=|++
  Torque for centripetal force : Fcn  Expr=sm.m_total*(u(1)^2+u(2)^2)/sm.l_boom*u(3)
  Trigonometric Function : Trigonometry
  Trunk Pitch Control : Fcn  Expr=ctrl.kp_torque_swing*(0-u(1)) + ctrl.kd_torque_swing*(0-u(2))
  Desired Stance Torques : Outport  OutputWhenDisabled=reset  InitialOutput=0
  wires:
  Selector2/1 -> Gain2/1
  Selector1/1 -> Gain1/1
  Sum4/1 -> Mux/3  "T_lat"
  Sum3/1 -> Sum4/2  "T_tipping"
  Gain1/1 -> Sum3/2
  Gain2/1 -> Sum3/1
  Torso Roll/1 -> Selector1/1, Selector2/1
  Torque for centripetal force/1 -> Sum4/1  "T_centripetal"
  Mux1/1 -> Torque for centripetal force/1
  z_torso/1 -> Mux1/3
  vx_torso/1 -> Mux1/1
  vz_torso/1 -> Mux1/2
  Selector/1 -> Demux/1
  Sum1/1 -> Mux/1  "T_b"
  Sum2/1 -> Mux/2  "T_f"
  Product/1 -> Sum2/2, Sum1/2
  Gain/1 -> Product/2
  Trigonometric Function/1 -> Gain/1
  Sum/1 -> Trigonometric Function/1
  Demux/2 -> Sum/2  "f"
  Demux/1 -> Sum/1  "b"
  Stance Leg Angle/1 -> Selector/1
  Constant/1 -> Product/1  "Leg force"
  Mux/1 -> Desired Stance Torques/1
  Trunk Pitch Control/1 -> Sum1/1, Sum2/1  "Leg torque"
  Torso Pitch/1 -> Trunk Pitch Control/1

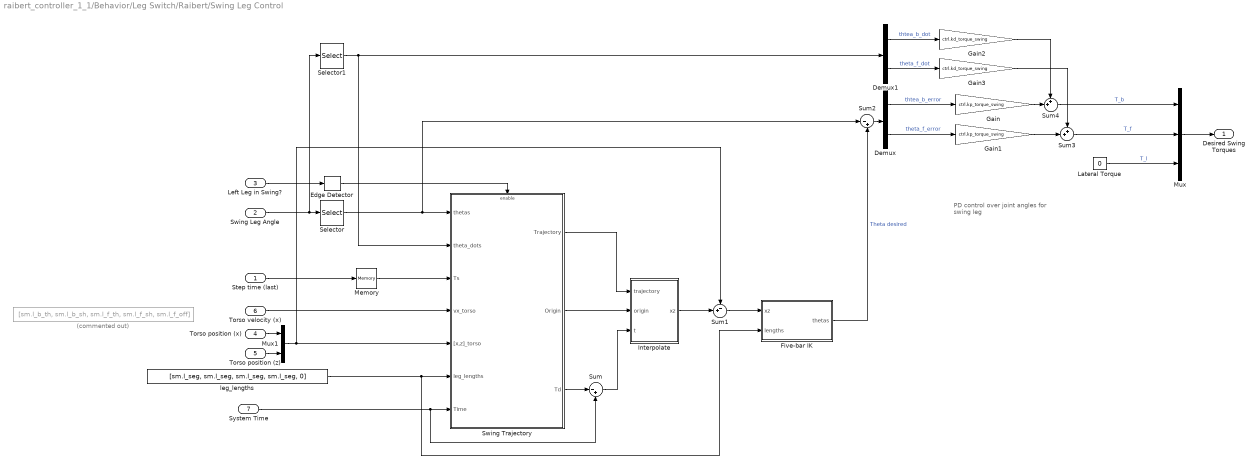
== system raibert_controller_1_1/Behavior/Leg Switch/Raibert/Swing Leg Control ==
  note: PD control over joint angles
      | for swing leg
  Step time (last) : Inport
  Swing Leg Angle : Inport  Port=2
  Left Leg in Swing? : Inport  Port=3
  Torso position (x) : Inport  Port=4
  Torso position (z) : Inport  Port=5
  Torso velocity (x) : Inport  Port=6
  System Time : Inport  Port=7
  " " : Constant  Commented=on  Value=[sm.l_b_th, sm.l_b_sh, sm.l_f_th, sm.l_f_sh, sm.l_f_off]
  " Lateral Torque" : Constant  Value=0
  Demux : Demux  Outputs=2
  Demux1 : Demux  Outputs=2
  Edge Detector : powerlib_meascontrol/Logic/Edge Detector  model=Either  ic=0  Ts=0
      settings: SourceProductName=Simscape Power Systems  SourceProductBaseCode=PS
  Five-bar IK : MATLAB Function  TreatAsAtomicUnit=on
  Gain : Gain  Gain=ctrl.kp_torque_swing
  Gain1 : Gain  Gain=ctrl.kp_torque_swing
  Gain2 : Gain  Gain=ctrl.kd_torque_swing
  Gain3 : Gain  Gain=ctrl.kd_torque_swing
  Interpolate : MATLAB Function  TreatAsAtomicUnit=on  SystemSampleTime=0.005
  Memory : Memory  InitialCondition=ctrl.stepping_time
  Mux : Mux  Inputs=3
  Mux1 : Mux  Inputs=2
  Selector : Selector  InputPortWidth=4  IndexOptions=Index vector (dialog)  Indices=[1 3]  OutputSizes=1
  Selector1 : Selector  InputPortWidth=4  IndexOptions=Index vector (dialog)  Indices=[2 4]  OutputSizes=1
  Sum : Sum  Inputs=|-+
  Sum1 : Sum  Inputs=-+|
  Sum2 : Sum  Inputs=|-+
  Sum3 : Sum  Inputs=++|
  Sum4 : Sum  Inputs=++|
  Swing Trajectory : Subsystem
  leg_lengths : Constant  Value=[sm.l_seg, sm.l_seg, sm.l_seg, sm.l_seg, 0]
  Desired Swing Torques : Outport  OutputWhenDisabled=reset  InitialOutput=0
  wires:
  Mux/1 -> Desired Swing Torques/1
  Edge Detector/1 -> Swing Trajectory/Enable
  " Lateral Torque"/1 -> Mux/3  "T_l"
  Gain3/1 -> Sum3/1
  Demux1/2 -> Gain3/1  "theta_f_dot"
  Gain1/1 -> Sum3/2
  Demux1/1 -> Gain2/1  "thtea_b_dot"
  Selector1/1 -> Demux1/1, Swing Trajectory/2(theta_dots)
  Selector/1 -> Swing Trajectory/1(thetas), Sum2/1
  Memory/1 -> Swing Trajectory/3(Ts)
  Sum3/1 -> Mux/2  "T_f"
  Sum4/1 -> Mux/1  "T_b"
  Gain2/1 -> Sum4/1
  Gain/1 -> Sum4/2
  Demux/2 -> Gain1/1  "theta_f_error"
  Sum2/1 -> Demux/1
  Demux/1 -> Gain/1  "thtea_b_error"
  Five-bar IK/1(thetas) -> Sum2/2  "Theta desired"
  Sum1/1 -> Five-bar IK/1(xz)
  Interpolate/1(xz) -> Sum1/2
  leg_lengths/1 -> Five-bar IK/2(lengths), Swing Trajectory/6(leg_lengths)
  Swing Trajectory/2(Origin) -> Interpolate/2(origin)
  Sum/1 -> Interpolate/3(t)
  Swing Trajectory/3(Td) -> Sum/1
  Swing Trajectory/1(Trajectory) -> Interpolate/1(trajectory)
  System Time/1 -> Sum/2, Swing Trajectory/7(Time)
  Swing Leg Angle/1 -> Selector/1, Selector1/1
  Mux1/1 -> Swing Trajectory/5("[x,z]_torso"), Sum1/1
  Torso position (z)/1 -> Mux1/2
  Torso position (x)/1 -> Mux1/1
  Torso velocity (x)/1 -> Swing Trajectory/4(vx_torso)
  Step time (last)/1 -> Memory/1
  Left Leg in Swing?/1 -> Edge Detector/1

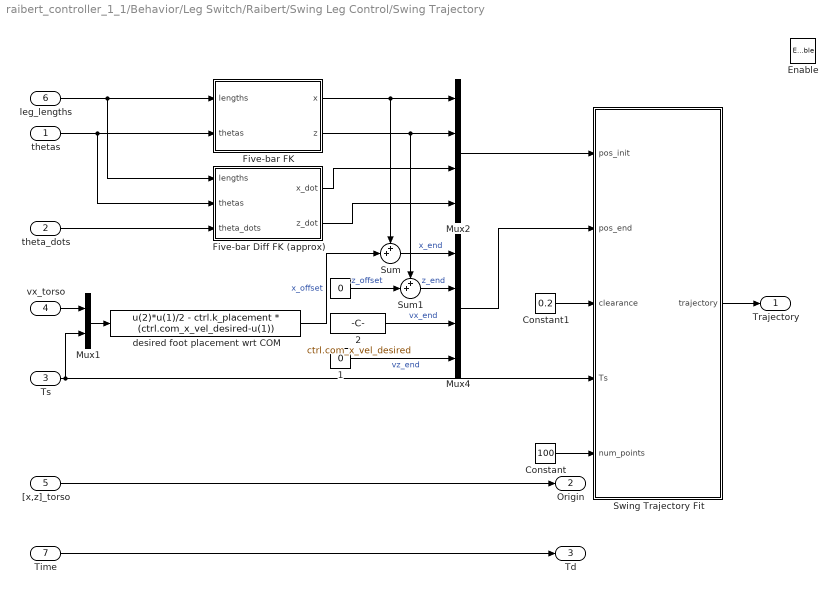
== system raibert_controller_1_1/Behavior/Leg Switch/Raibert/Swing Leg Control/Swing Trajectory ==
  thetas : Inport
  theta_dots : Inport  Port=2
  Ts : Inport  Port=3
  vx_torso : Inport  Port=4
  "[x,z]_torso" : Inport  Port=5
  leg_lengths : Inport  Port=6
  Time : Inport  Port=7
  Enable : EnablePort  PropagateVarSize=During execution
  " " : Constant  Value=0
  " 1" : Constant  Value=0
  " 2" : Constant  Value=ctrl.com_x_vel_desired
  Constant : Constant  Value=100
  Constant1 : Constant  Value=0.2
  Five-bar Diff FK (approx) : MATLAB Function  TreatAsAtomicUnit=on
  Five-bar FK : MATLAB Function  TreatAsAtomicUnit=on
  Mux1 : Mux  Inputs=2
  Mux2 : Mux
  Mux4 : Mux
  Sum : Sum  Inputs=++|
  Sum1 : Sum  Inputs=++|
  Swing Trajectory Fit : MATLAB Function  TreatAsAtomicUnit=on  SystemSampleTime=0.005
  desired foot placement wrt COM : Fcn  Expr=u(2)*u(1)/2 - ctrl.k_placement * (ctrl.com_x_vel_desired-u(1))
  Trajectory : Outport
  Origin : Outport  Port=2
  Td : Outport  Port=3
  wires:
  theta_dots/1 -> Five-bar Diff FK (approx)/3(theta_dots)
  " 2"/1 -> Mux4/3  "vx_end"
  " 1"/1 -> Mux4/4  "vz_end"
  Mux4/1 -> Swing Trajectory Fit/2(pos_end)
  Sum1/1 -> Mux4/2  "z_end"
  Sum/1 -> Mux4/1  "x_end"
  Five-bar Diff FK (approx)/2(z_dot) -> Mux2/4
  Five-bar Diff FK (approx)/1(x_dot) -> Mux2/3
  thetas/1 -> Five-bar FK/2(thetas), Five-bar Diff FK (approx)/2(thetas)
  Time/1 -> Td/1
  leg_lengths/1 -> Five-bar FK/1(lengths), Five-bar Diff FK (approx)/1(lengths)
  Mux2/1 -> Swing Trajectory Fit/1(pos_init)
  Five-bar FK/2(z) -> Mux2/2, Sum1/1
  Five-bar FK/1(x) -> Mux2/1, Sum/1
  "[x,z]_torso"/1 -> Origin/1
  " "/1 -> Sum1/2  "z_offset"
  desired foot placement wrt COM/1 -> Sum/2  "x_offset"
  vx_torso/1 -> Mux1/1
  Mux1/1 -> desired foot placement wrt COM/1
  Constant1/1 -> Swing Trajectory Fit/3(clearance)
  Constant/1 -> Swing Trajectory Fit/5(num_points)
  Ts/1 -> Mux1/2, Swing Trajectory Fit/4(Ts)
  Swing Trajectory Fit/1(trajectory) -> Trajectory/1

== matlab function raibert_controller_1_1/Behavior/Leg Switch/Raibert/Swing Leg Control/Five-bar IK ==
  data: xz input; thetas output; lengths input
function thetas = fcn(xz,lengths)
    % thetas - [theta_b, theta_f] in range [0,2*pi]
    % lengths - [l_b_th, l_b_sh, l_f_th, l_f_sh, l_f_off]
    l1 = lengths(1); % l_b_th
    l2 = lengths(2); % l_b_sh
    l3 = lengths(3); % l_f_th
    l4 = lengths(4); % l_f_sh
    l5 = lengths(5); % l_f_off
    
    x = xz(1);
    z = xz(2);
    thetas = [0,0];
    theta_foot = atan2(z,x);
    if (theta_foot < 0)
        theta_foot = theta_foot + 2*pi;
    end
    d_foot = sqrt(x^2+z^2);
    assert(abs((d_foot^2 + l3^2 - (l4+l5)^2)/(2*d_foot*l3))<=1, 'Check Swing Trajectory!');
    thetas(2) = theta_foot + acos((d_foot^2 + l3^2 - (l4+l5)^2)/(2*d_foot*l3));
    
    theta_knee_f = pi + acos((l3^2 + (l4+l5)^2 - (x^2+z^2))/(2*l3*(l4+l5)));
    x_ankle = x - l5*cos(theta_knee_f + thetas(2));
    z_ankle = z - l5*sin(theta_knee_f + thetas(2));
    theta_ankle = atan2(z_ankle,x_ankle);
    if (theta_ankle < 0)
        theta_ankle = theta_ankle + 2*pi;
    end
    d_ankle = sqrt(x_ankle^2+z_ankle^2);
    assert(abs((d_ankle^2 + l1^2 - l2^2)/(2*d_ankle*l1))<=1, 'Check Swing Trajectory!');
    thetas(1) = theta_ankle - acos((d_ankle^2 + l1^2 - l2^2)/(2*d_ankle*l1));
end

== matlab function raibert_controller_1_1/Behavior/Leg Switch/Raibert/Swing Leg Control/Interpolate ==
  data: trajectory input; origin input; xz output; t input
function xz = fcn(trajectory, origin, t)
    if (t>trajectory(end,1))
        xz = trajectory(end,2:3);
    else
        xz = zeros(1,2);
        xz(1) = interp1(trajectory(:,1), trajectory(:,2), t);
        xz(2) = interp1(trajectory(:,1), trajectory(:,3), t);
    end
    xz(1) = xz(1) + origin(1);
    xz(2) = xz(2) + origin(2);
end

== matlab function raibert_controller_1_1/Behavior/Leg Switch/Raibert/Swing Leg Control/Swing Trajectory/Five-bar Diff FK (approx) ==
  data: x_dot output; lengths input; z_dot output; thetas input; theta_dots input
function [x_dot,z_dot] = fcn(lengths, thetas, theta_dots)
    % theta - [theta_b, theta_f]
    % lengths - [l_b_th, l_b_sh, l_f_th, l_f_sh, l_f_off]
    l1 = lengths(1); % l_b_th
    l2 = lengths(2); % l_b_sh
    l3 = lengths(3); % l_f_th
    l4 = lengths(4); % l_f_sh
    l5 = lengths(5); % l_f_off
    
    assert(thetas(2) > thetas(1), sprintf('Front angle(%f) < Back angle(%f)',thetas(2),thetas(1)));
    
    l = 0.25*(l1+l2+l3+l4);
    
%     v_par = -l*sin((thetas(2) - thetas(1))/2)*(theta_dots(2) - theta_dots(1));
%     v_perp = l*cos((thetas(2) - thetas(1))/2)*(theta_dots(2) + theta_dots(1));
    
    x_dot = -l*theta_dots(1)*sin(thetas(1)) - l*theta_dots(2)*sin(thetas(2));
    z_dot = l*theta_dots(1)*cos(thetas(1)) + l*theta_dots(2)*cos(thetas(2));
    
end

== matlab function raibert_controller_1_1/Behavior/Leg Switch/Raibert/Swing Leg Control/Swing Trajectory/Five-bar FK ==
  data: x output; lengths input; z output; thetas input
function [x,z] = fcn(lengths, thetas)
    % theta - [theta_b, theta_f]
    % lengths - [l_b_th, l_b_sh, l_f_th, l_f_sh, l_f_off]
    l1 = lengths(1); % l_b_th
    l2 = lengths(2); % l_b_sh
    l3 = lengths(3); % l_f_th
    l4 = lengths(4); % l_f_sh
    l5 = lengths(5); % l_f_off
    
    assert(thetas(2) > thetas(1), sprintf('Front angle(%f) < Back angle(%f)',thetas(2),thetas(1)));
    
    x_knee_b = l1*cos(thetas(1));
    z_knee_b = l1*sin(thetas(1));
    
    x_knee_f = l3*cos(thetas(2));
    z_knee_f = l3*sin(thetas(2));
    
    theta_hip = thetas(2) - thetas(1);
    theta_ankle = acos((l2^2 + l4^2 - ((x_knee_b-x_knee_f)^2 + (z_knee_b-z_knee_f)^2))/(2*l2*l4));
    
    % 2pi - theta_hip - theta_ankle = theta_knee_f + theta_knee_b
    % l_f_th^2 + l_f_sh^2 - 2(l_f_th)(l_f_sh)cos(theta_knee_f) = l_b_th^2 + l_b_sh^2 - 2(l_b_th)(l_b_sh)cos(theta_knee_b)
    c = 2*pi -theta_hip - theta_ankle;
    alpha = atan2(-l3*l4*sin(c),l1*l2-l3*l4*cos(c));
    if (alpha<0)
        alpha = 2*pi+alpha;
    end
    
    theta_1 = acos((l3^2 + l4^2 - l1^2 - l2^2)/(2*sqrt((l3*l4*sin(c))^2+(l1*l2-l3*l4*cos(c))^2)));
    theta_knee_f1 = alpha + theta_1;
    theta_knee_f2 = alpha - theta_1;
    
    if (theta_knee_f1 > 2*pi)
        theta_knee_f1 = theta_knee_f1 - 2*pi;
    end

    if (theta_knee_f2 < 0)
        theta_knee_f2 = theta_knee_f2 + 2*pi;
    end
    
    if ((theta_knee_f1 > 0) && ((c - theta_knee_f1) > 0))
        theta_knee_f = theta_knee_f1+pi;
    elseif((theta_knee_f2 > 0) && ((c - theta_knee_f2) > 0))
        theta_knee_f = theta_knee_f2+pi;
    else
        theta_knee_f = min(abs(theta_knee_f1), abs(theta_knee_f2));
    end
    
   x = x_knee_f + (l4+l5)*cos(theta_knee_f + thetas(2));
   z = z_knee_f + (l4+l5)*sin(theta_knee_f + thetas(2));
    
end

== matlab function raibert_controller_1_1/Behavior/Leg Switch/Raibert/Swing Leg Control/Swing Trajectory/Swing Trajectory Fit ==
  data: pos_init input; trajectory output size=[100 3]; pos_end input; clearance input; Ts input; num_points input
function trajectory = fcn(pos_init, pos_end, clearance, Ts, num_points)
    
    t_points = [0,Ts/2,Ts];
    x_points = [pos_init(1), (pos_init(1) + pos_end(1))/2, pos_end(1)];
    z_points = [pos_init(2), clearance+(pos_init(2) + pos_end(2))/2, pos_end(2)];
    
    t_q = linspace(0,Ts,num_points);
%     x_spline = csape(t_points, x_points, 'complete', [pos_init(3), pos_end(3)]);
%     z_spline = csape(t_points, z_points, 'complete', [pos_init(4), pos_end(4)]);
    x_spline = spline(t_points, x_points, t_q);
    z_spline = spline(t_points, z_points, t_q);
    
%     trajectory = [t_q', fnval(x_spline, tq)', fnval(z_spline, tq)'];
    trajectory = [t_q', x_spline', z_spline'];
    
%     l_th_f = 0.5;
%     l_th_b = 0.5;
%     l_sh_f = 0.4;
%     l_sh_b = 0.4;
%     l_sh_off = 0.15;
%     for i=1:1:size(traj,1)
%         x = traj(i,1);
%         y = traj(i,2);
%         theta_th_f = acos(x/sqrt(x^2+y^2)) - acos((x^2 + y^2 + l_th_f^2 - (l_sh_f+l_sh_off)^2)/((2*l_th_f)*(sqrt(x^2+y^2))));
%     end
    
end

== matlab function raibert_controller_1_1/Behavior/Convert to Body Frame IMU Accelerations ==
  data: accelerometer input; imu_accelerations output
function imu_accelerations = imu_to_body_frame(accelerometer)
    g = 9.803;
    z_up_rotation = [1, 0, 0; 0, 0, 1; 0, -1, 0];
    align_xy_rotation = [sqrt(2)/2, -sqrt(2)/2, 0; sqrt(2)/2, sqrt(2)/2, 0; 0, 0, 1];
    imu_accelerations = g*z_up_rotation*align_xy_rotation*accelerometer;
end
